simulink model "feedback"  (Simulink 7.6)
settings: Solver=FixedStepDiscrete  StartTime=0.0  StopTime=10.0  FixedStep=0.001  RelTol=1e-3
undefined symbols (not defined in the file): denlow, numlow
libraries: simulink x1
settings Model: Creator=Fodi  LastModifiedBy=Fodi

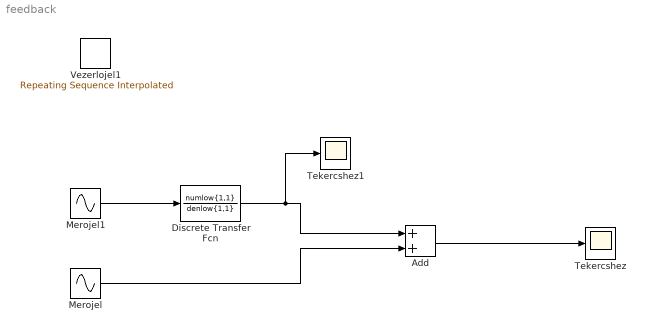
== system feedback ==
  Add : Sum
  Discrete Transfer Fcn : DiscreteTransferFcn  Numerator=numlow{1,1}  Denominator=denlow{1,1}  SampleTime=0.001
  Merojel : Sin  SampleTime=0.001
  Merojel1 : Sin  Frequency=100  SampleTime=0.001
  Tekercshez : Scope
  Tekercshez1 : Scope
      settings: TimeRange=10  YMin=-2e+305  YMax=1.2e+306
  Vezerlojel1 : simulink/Sources/Repeating Sequence Interpolated  SystemSampleTime=-1  OutValues=[3 1 4 2 1].'  TimeValues=[0 0.1 0.5 0.6 1].'  LookUpMeth=Interpolation-Use End Values  tsamp=0.001  OutMin=[]  OutMax=[]  OutDataTypeStr=double  OutputDataTypeScalingMode=double  OutDataType=fixdt(0,8)  OutScaling=2^-10
  wires:
  Merojel1/1 -> Discrete Transfer Fcn/1
  Discrete Transfer Fcn/1 -> Add/1, Tekercshez1/1
  Merojel/1 -> Add/2
  Add/1 -> Tekercshez/1
